simulink model "control_att_INDI"  (R2021a)
settings: Solver=FixedStepAuto  StartTime=0.0  StopTime=10.0  RelTol=1e-3
undefined symbols (not defined in the file or in its folder): par
libraries: eeGeneralControl x7, simulink x4
settings Model: Creator=root  LastModifiedBy=root

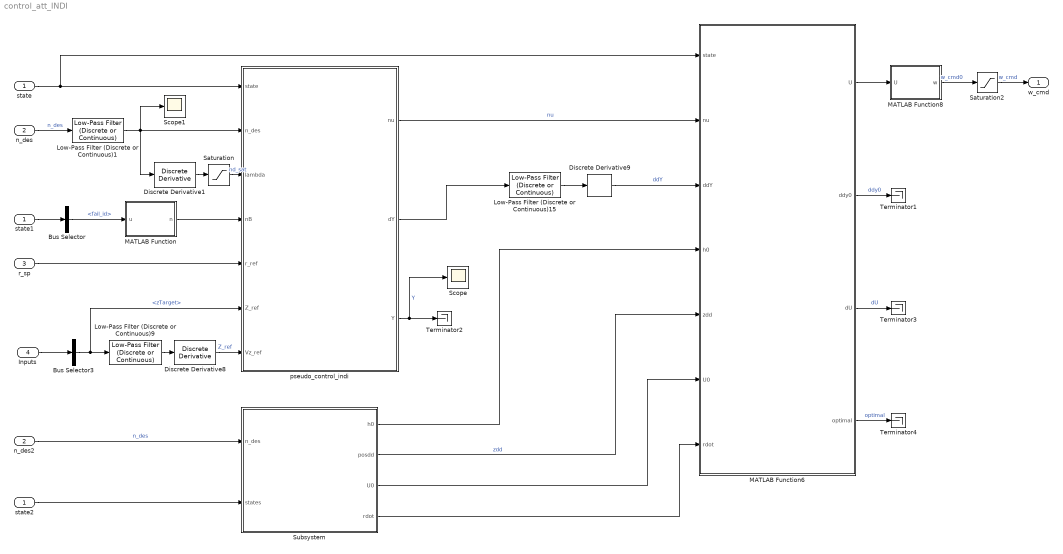
== system control_att_INDI ==
  state : Inport  OutDataTypeStr=Bus:stateBus
  n_des : Inport  Port=2  PortDimensions=3
  r_sp : Inport  Port=3
  Inputs : Inport  Port=4  OutDataTypeStr=Bus:inputsBus
  Bus Selector : BusSelector  OutputSignals=fail_id
  Bus Selector3 : BusSelector  OutputSignals=zTarget
  Discrete Derivative1 : simulink/Discrete/Discrete Derivative  gainval=1.0  ICPrevScaledInput=0.0  OutMin=[]  OutMax=[]  OutDataType=fixdt(1, 16)  OutScaling=2^-10  DoSatur=off
  Discrete Derivative8 : simulink/Discrete/Discrete Derivative  gainval=1.0  ICPrevScaledInput=0.0  OutMin=[]  OutMax=[]  OutDataType=fixdt(1, 16)  OutScaling=2^-10  DoSatur=off
  Discrete Derivative9 : simulink/Discrete/Discrete Derivative  gainval=1.0  ICPrevScaledInput=0.0  OutMin=[]  OutMax=[]  OutDataType=fixdt(1, 16)  OutScaling=2^-10  DoSatur=off
  Low-Pass Filter (Discrete or Continuous)1 : eeGeneralControl/Low-Pass Filter (Discrete or Continuous)  K=1  T=par.t_indi  B=inf  A=-inf  init_option=Inherited from block input  x0=0  Ts=-1
  Low-Pass Filter (Discrete or Continuous)15 : eeGeneralControl/Low-Pass Filter (Discrete or Continuous)  K=1  T=par.t_indi  B=inf  A=-inf  init_option=Inherited from block input  x0=0  Ts=-1
  Low-Pass Filter (Discrete or Continuous)9 : eeGeneralControl/Low-Pass Filter (Discrete or Continuous)  K=1  T=par.t_indi  B=inf  A=-inf  init_option=Inherited from block input  x0=0  Ts=-1
  MATLAB Function : MATLAB Function  TreatAsAtomicUnit=on
  MATLAB Function6 : MATLAB Function  TreatAsAtomicUnit=on
  MATLAB Function8 : MATLAB Function  TreatAsAtomicUnit=on
  Saturation : Saturate
  Saturation2 : Saturate  UpperLimit=par.w_max  LowerLimit=par.w_min
  Scope : Scope
  Scope1 : Scope
  Subsystem : Subsystem
  Terminator{1..4} (4 alike) : Terminator
  n_des2 : InportShadow  Port=2  PortDimensions=3
  pseudo_control_indi : MATLAB Function  TreatAsAtomicUnit=on
  state1 : InportShadow  OutDataTypeStr=Bus:stateBus
  state2 : InportShadow  OutDataTypeStr=Bus:stateBus
  w_cmd : Outport  VectorParamsAs1DForOutWhenUnconnected=off
  wires:
  MATLAB Function6/4(optimal) -> Terminator4/1  "optimal"
  Inputs/1 -> Bus Selector3/1
  Bus Selector3/1 -> Low-Pass Filter (Discrete or Continuous)9/1, pseudo_control_indi/6(Z_ref)  "<zTarget>"
  n_des2/1 -> Subsystem/1(n_des)  "n_des"
  Subsystem/1(h0) -> MATLAB Function6/4(h0)
  Low-Pass Filter (Discrete or Continuous)9/1 -> Discrete Derivative8/1
  Saturation2/1 -> w_cmd/1  "w_cmd"
  Discrete Derivative9/1 -> MATLAB Function6/3(ddY)  "ddY"
  MATLAB Function/1(n) -> pseudo_control_indi/4(nB)
  n_des/1 -> Low-Pass Filter (Discrete or Continuous)1/1  "n_des"
  Subsystem/2(posdd) -> MATLAB Function6/5(zdd)  "zdd"
  MATLAB Function6/2(ddy0) -> Terminator1/1  "ddy0"
  Low-Pass Filter (Discrete or Continuous)15/1 -> Discrete Derivative9/1
  MATLAB Function6/1(U) -> MATLAB Function8/1(U)
  r_sp/1 -> pseudo_control_indi/5(r_ref)
  Bus Selector/1 -> MATLAB Function/1(u)  "<fail_id>"
  Discrete Derivative1/1 -> Saturation/1
  pseudo_control_indi/3(Y) -> Scope/1, Terminator2/1  "Y"
  pseudo_control_indi/2(dY) -> Low-Pass Filter (Discrete or Continuous)15/1
  Saturation/1 -> pseudo_control_indi/3(lambda)  "nd_sat"
  state/1 -> pseudo_control_indi/1(state), MATLAB Function6/1(state)
  MATLAB Function6/3(dU) -> Terminator3/1  "dU"
  Discrete Derivative8/1 -> pseudo_control_indi/7(Vz_ref)  "Z_ref"
  Subsystem/3(U0) -> MATLAB Function6/6(U0)
  state2/1 -> Subsystem/2(states)
  state1/1 -> Bus Selector/1
  Low-Pass Filter (Discrete or Continuous)1/1 -> Scope1/1, Discrete Derivative1/1, pseudo_control_indi/2(n_des)
  Subsystem/4(rdot) -> MATLAB Function6/7(rdot)
  pseudo_control_indi/1(nu) -> MATLAB Function6/2(nu)  "nu"
  MATLAB Function8/1(w) -> Saturation2/1  "w_cmd0"

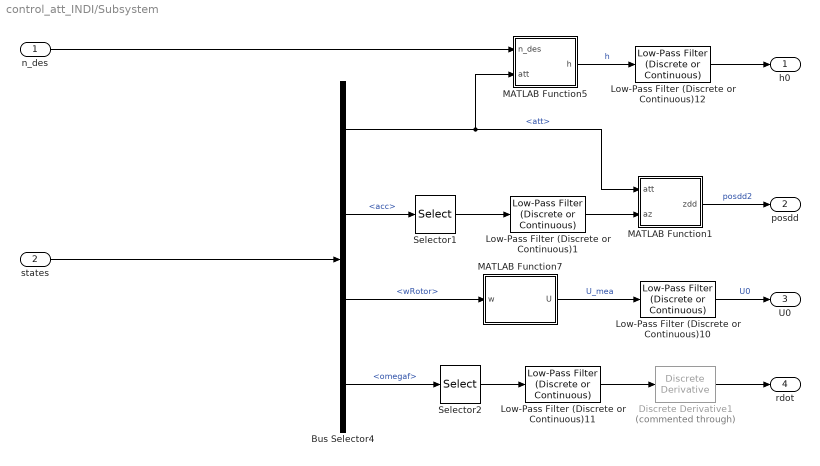
== system control_att_INDI/Subsystem ==
  n_des : Inport
  states : Inport  Port=2
  Bus Selector4 : BusSelector  OutputSignals=att,acc,wRotor,omegaf
  Discrete Derivative1 : simulink/Discrete/Discrete Derivative  Commented=through  gainval=1.0  ICPrevScaledInput=0.0  OutMin=[]  OutMax=[]  OutDataType=fixdt(1, 16)  OutScaling=2^-10  DoSatur=off
  Low-Pass Filter (Discrete or Continuous){1,10..12} (4 alike) : eeGeneralControl/Low-Pass Filter (Discrete or Continuous)  K=1  T=par.t_indi  B=inf  A=-inf  init_option=Inherited from block input  x0=0  Ts=-1
  MATLAB Function1 : MATLAB Function  TreatAsAtomicUnit=on
  MATLAB Function5 : MATLAB Function  TreatAsAtomicUnit=on
  MATLAB Function7 : MATLAB Function  TreatAsAtomicUnit=on
  Selector1 : Selector  InputPortWidth=3  IndexOptions=Index vector (dialog)  Indices=3  OutputSizes=1
  Selector2 : Selector  InputPortWidth=3  IndexOptions=Index vector (dialog)  Indices=3  OutputSizes=1
  h0 : Outport  VectorParamsAs1DForOutWhenUnconnected=off
  posdd : Outport  Port=2  VectorParamsAs1DForOutWhenUnconnected=off
  U0 : Outport  Port=3  VectorParamsAs1DForOutWhenUnconnected=off
  rdot : Outport  Port=4  VectorParamsAs1DForOutWhenUnconnected=off
  wires:
  MATLAB Function1/1(zdd) -> posdd/1  "posdd2"
  Low-Pass Filter (Discrete or Continuous)1/1 -> MATLAB Function1/2(az)
  Selector1/1 -> Low-Pass Filter (Discrete or Continuous)1/1
  Bus Selector4/2 -> Selector1/1  "<acc>"
  n_des/1 -> MATLAB Function5/1(n_des)
  Low-Pass Filter (Discrete or Continuous)12/1 -> h0/1
  Low-Pass Filter (Discrete or Continuous)11/1 -> Discrete Derivative1/1
  Low-Pass Filter (Discrete or Continuous)10/1 -> U0/1  "U0"
  MATLAB Function7/1(U) -> Low-Pass Filter (Discrete or Continuous)10/1  "U_mea"
  Selector2/1 -> Low-Pass Filter (Discrete or Continuous)11/1
  MATLAB Function5/1(h) -> Low-Pass Filter (Discrete or Continuous)12/1  "h"
  states/1 -> Bus Selector4/1
  Bus Selector4/1 -> MATLAB Function1/1(att), MATLAB Function5/2(att)  "<att>"
  Bus Selector4/3 -> MATLAB Function7/1(w)  "<wRotor>"
  Bus Selector4/4 -> Selector2/1  "<omegaf>"
  Discrete Derivative1/1 -> rdot/1

== matlab function control_att_INDI/MATLAB Function ==
  data: u input; n output; par parameter
function n = fcn(u,par)

a = par.axis_tilt;

if par.DRF_enable == 0 || par.DRF_enable == 1 
    if u == 1
       n = [-a, a, -1];   
    elseif u == 2
       n = [-a, -a, -1];
    elseif u == 3
       n = [a, -a, -1];
    elseif u == 4
       n = [a, a, -1];
    else
       n = [0, 0, -1];    
    end
else
   n = [0, 0, -1];
end

== matlab function control_att_INDI/MATLAB Function6 ==
  data: state input; nu input; ddY input; h0 input; zdd input; U0 input; rdot input; U output; par parameter; ddy0 output; dU output; optimal output
function [U,ddy0,dU, optimal]  =  allocation_att_indi(state, nu, ddY, h0, zdd, U0, rdot, par)

ddy0 = zeros(4,2);
if par.allocType == 1
    [U,ddy0(:,1),dU]  =  allocation_att_indi(state, nu, ddY, h0, zdd, U0, rdot, par);
    optimal = [1 0];
elseif par.allocType == 2
    [U,ddy0, dU, optimal]  =  allocation_qpindi(state, nu, ddY, h0, zdd, U0, rdot, par);
else
    error('invalide allocation method');
end
end

== matlab function control_att_INDI/Subsystem/MATLAB Function1 ==
  data: att input; az input; zdd output
function zdd = fcn(att,az)

phi = att(1);
theta = att(2);

zdd = az*cos(theta)*cos(phi) + 9.8124;

== matlab function control_att_INDI/MATLAB Function8 ==
  data: U input; w output
function w = U2omega(U)
%#codegen

w = zeros(4,1);
w(1) = sqrt(abs(U(1)))*sign(U(1));
w(2) = sqrt(abs(U(2)))*sign(U(2));
w(3) = sqrt(abs(U(3)))*sign(U(3));
w(4) = sqrt(abs(U(4)))*sign(U(4));

end

== matlab function control_att_INDI/Subsystem/MATLAB Function5 ==
  data: n_des input; att input; h output
function h = fcn(n_des, att)

phi = att(1);
theta = att(2);
psi = att(3);

R_IB = euler2Rot(phi,theta,psi);

h = R_IB \ n_des;

== matlab function control_att_INDI/Subsystem/MATLAB Function7 ==
  data: w input; U output
function U = omega2U(w)
%#codegen

U = zeros(4,1);
U(1) = w(1)^2;
U(2) = w(2)^2;
U(3) = w(3)^2;
U(4) = w(4)^2;
end

== matlab function control_att_INDI/pseudo_control_indi ==
  data: state input; n_des input; lambda input; nB input; r_ref input; Z_ref input; Vz_ref input; nu output; par parameter; dY output; Y output
function [nu,dY, Y] = pseudo_control_att_indi(state, n_des, lambda, nB, r_ref, Z_ref, Vz_ref, par)

[nu, dY, Y] = pseudo_control_att_indi(state, n_des, lambda, nB, r_ref, Z_ref, Vz_ref, par);

end
